simulink model "testHinfControlOutputFeedback"  (R2023b)
settings: Solver=ode1  StartTime=0.0  StopTime=20  FixedStep=h/10000  RelTol=1e-3
values from neighbouring files (symbols this model uses):
  A = [0 1 ; -1 0]    [DLMI_code_validation.m]    (also in DLMI_translational_controller_design.m = [    0           1         zeros(1,2)         0        zeros; DLQR_rotational_controller_design.m = min_sys.A; DLQR_translational_controller.m = [-a3_ss -a2_ss -a1_ss -a0_ss b2_ss b1_ss b0_ss; discretization_with_delay.m = [Ad Bd1; zeros(1,size(Ad,2)) 0])
  A_hat_r = rsys.A    [DLMI_translational_controller_design.m]
  B = [0 ; 1]    [DLMI_code_validation.m]    (also in DLMI_translational_controller_design.m = [0 ; (1/m)*Dmd*Dm ; zeros(2,1) ; Bm ; Bmd*Dm]; DLQR_rotational_controller_design.m = min_sys.B; DLQR_translational_controller.m = [b3_ss ; 0 ; 0 ; 0 ; 1 ; 0 ; 0]; discretization_with_delay.m = [Bd2 ; 1])
  B_hat_r = rsys.B    [DLMI_translational_controller_design.m]
  C_hat_r = rsys.C    [DLMI_translational_controller_design.m]
  Cc = [1 0 ; 0 0]    [DLMI_code_validation.m]    (also in DLMI_translational_controller_design.m = [1 0 zeros(1,2) 0 zeros(1,2)])
  Cd = [1 ; 0]'    [DLMI_code_validation.m]    (also in DLMI_translational_controller_design.m = [Ds 0 Cs 0 zeros(1,2)])
  D_hat_r = rsys.D    [DLMI_translational_controller_design.m]
  Dc = [0 ; d]    [DLMI_code_validation.m]    (also in DLMI_translational_controller_design.m = 0)
  Ec = B    [DLMI_code_validation.m]    (also in DLMI_translational_controller_design.m = [0 ; (1/m) ; zeros(2,1)  ; 0 ; zeros(2,1)])
  h = 0.125    [Controllers_Design.m]    (also in DLMI_code_validation.m = 1; DLQR_rotational_controller_design.m = Pc_inv(end,:); DLQR_translational_controller.m = Pc_inv(end,:))
  omega = array_omega(index_omega)    [DLMI_translational_controller_design.m]
settings Model: Creator=Kawakami  LastModifiedBy=Luan

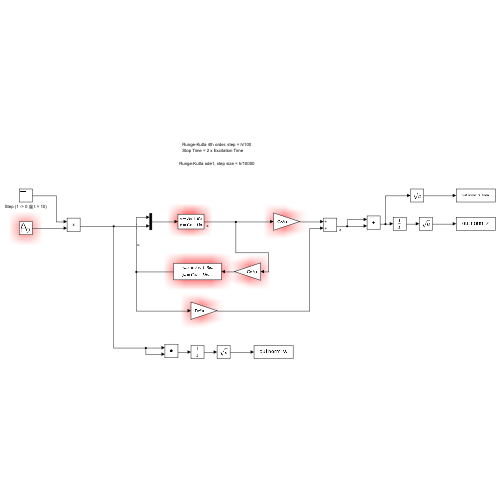
[thumbnail: Simulink's stored preview of the top-level diagram]
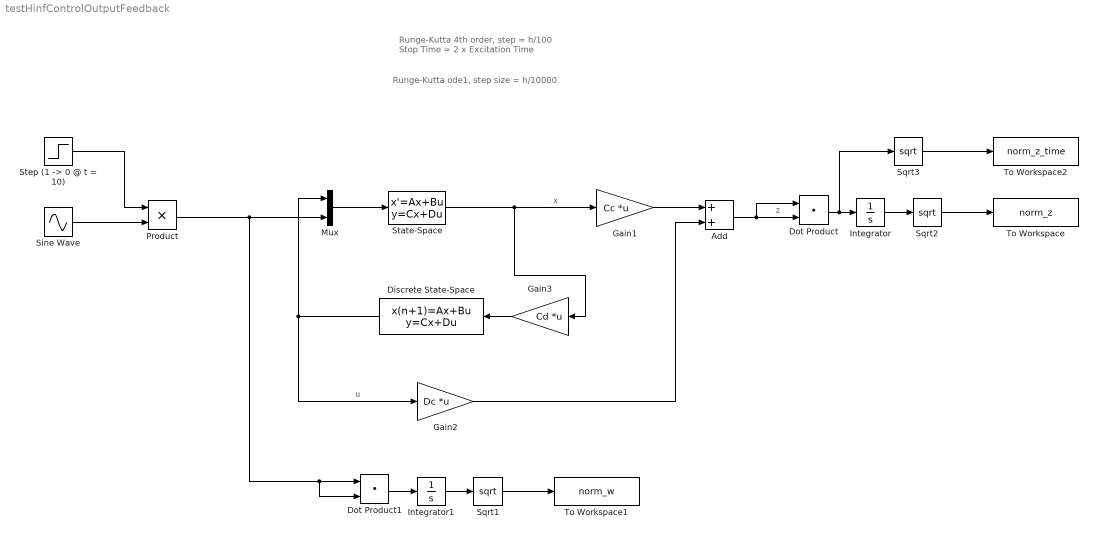
== system testHinfControlOutputFeedback ==
  note: Runge-Kutta ode1, step size = h/10000
  note: Runge-Kutta 4th order, step = h/100
      | Stop Time = 2 x Excitation Time
  Add : Sum
  Discrete State-Space : DiscreteStateSpace  A=A_hat_r  B=B_hat_r  C=C_hat_r  D=D_hat_r  InitialCondition=zeros(size(A_hat_r,1),1)  SampleTime=h
  Dot Product : DotProduct  OutDataTypeStr=Inherit: Inherit via internal rule
  Dot Product1 : DotProduct  OutDataTypeStr=Inherit: Inherit via internal rule
  Gain1 : Gain  Gain=Cc  Multiplication=Matrix(K*u)
  Gain2 : Gain  Gain=Dc  Multiplication=Matrix(K*u)
  Gain3 : Gain  Gain=Cd  Multiplication=Matrix(K*u)
  Integrator : Integrator
  Integrator1 : Integrator
  Mux : Mux  Inputs=2
  Product : Product
  Sine Wave : Sin  Frequency=omega  SampleTime=0
  Sqrt1 : Sqrt
  Sqrt2 : Sqrt
  Sqrt3 : Sqrt
  State-Space : StateSpace  A=A  B=[B Ec]  C=eye(size(A,1))  D=zeros(size(A,1),2)  InitialCondition=0
  "Step (1 -> 0 @ t = 10)" : Step  Time=10  Before=1  After=0  SampleTime=0
  To Workspace : ToWorkspace  VariableName=norm_z  SampleTime=-1
      settings: MaxDataPoints=1
  To Workspace1 : ToWorkspace  VariableName=norm_w  SampleTime=-1
      settings: MaxDataPoints=1
  To Workspace2 : ToWorkspace  VariableName=norm_z_time  SampleTime=-1
  wires:
  Mux/1 -> State-Space/1
  Discrete State-Space/1 -> Mux/1, Gain2/1  "u"
  State-Space/1 -> Gain3/1, Gain1/1  "x"
  Gain1/1 -> Add/1
  Gain2/1 -> Add/2
  Add/1 -> Dot Product/1, Dot Product/2  "z"
  Dot Product/1 -> Sqrt3/1, Integrator/1
  Integrator/1 -> Sqrt2/1
  Sqrt2/1 -> To Workspace/1
  Sqrt1/1 -> To Workspace1/1
  Integrator1/1 -> Sqrt1/1
  Dot Product1/1 -> Integrator1/1
  Sine Wave/1 -> Product/2
  "Step (1 -> 0 @ t = 10)"/1 -> Product/1
  Product/1 -> Dot Product1/2, Dot Product1/1, Mux/2
  Sqrt3/1 -> To Workspace2/1
  Gain3/1 -> Discrete State-Space/1
